simulink model "part1"  (R2020a)
settings: Solver=VariableStepAuto  StartTime=0.0  StopTime=3000  RelTol=1e-3
undefined symbols (not defined in the file): ConstSPSuge, ConstSPSway, ConstSPYaw, Current_input_type, Current_Speed, CurrHead, Hoerner, Kd_surge, Kd_sway, Kd_yaw, Ki_surge, Ki_sway, Ki_yaw, Kp_surge, Kp_sway, Kp_yaw, typeOfSimulation, vessel
libraries: marine_gnc x5, simulink x1, marine_hydro x1
settings Model: Creator=jonbjor  LastModifiedBy=joach
settings DataIOCC: ReturnWorkspaceOutputs=off
settings DebuggingCC: ArithmeticOperatorsInVariantConditions=warning
settings SFSimCC: SimUseLocalCustomCode=off  CustomCodeUndefinedFunction=UseInterfaceOnly
settings RTWCC: RTWUseLocalCustomCode=off

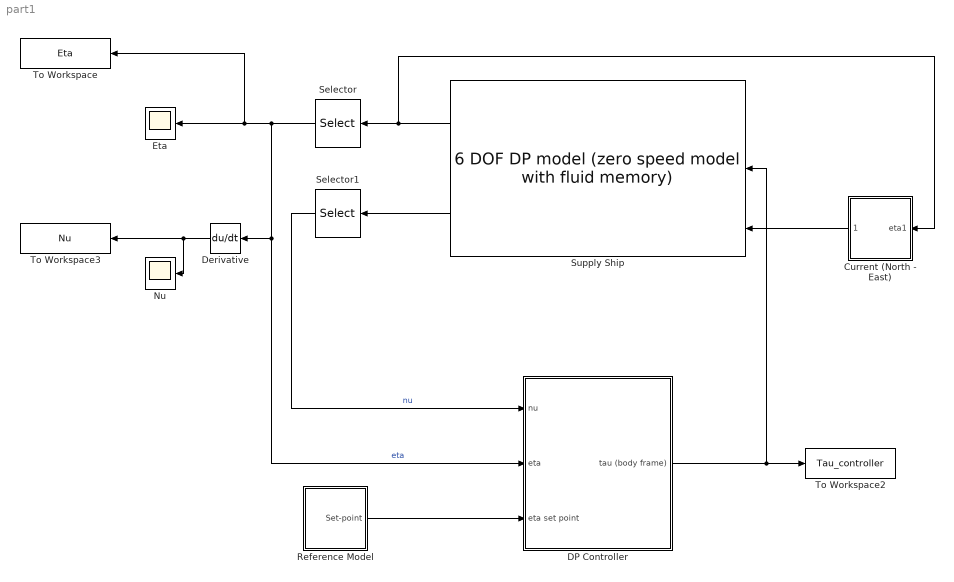
== system part1 ==
  Current (North - East) : Subsystem
  DP Controller : Subsystem
  Derivative : Derivative
  Eta : Scope
  Nu : Scope
  Reference Model : Subsystem
  Selector : Selector  InputPortWidth=6  IndexOptions=Index vector (dialog)  Indices=[1 2 6]  OutputSizes=1
  Selector1 : Selector  InputPortWidth=6  IndexOptions=Index vector (dialog)  Indices=[1 2 6]  OutputSizes=1
  Supply Ship : marine_hydro/Hydro Library/6 DOF DP model  (zero speed model with fluid memory)  ABC=vesselABC  rho=1025  Axc=0.9*vessel.main.T*vessel.main.B  Ayc=0.9*vessel.main.T*vessel.main.Lpp  CX=1  CY_2D=Hoerner(vessel.main.B,vessel.main.T)  Bv=vessel.Bv  mask(6 DOF zero speed model){}
      link override "Integrator1 ": InitialCondition=nu0
      link override Integrator2: InitialCondition=eta0
      settings: SourceProductName=MSS Hydro
      mask Display:
      | image('supply.jpg');
      | color('white'); port_label('output', 1, 'eta')
      | color('white'); port_label('output', 2, 'nu')
      | color('white'); port_label('input', 1, 'tau_wave')
      | color('white'); port_label('input', 2, 'tau')
      | color('white'); port_label('input', 3, 'nu_c')
  To Workspace : ToWorkspace  VariableName=Eta  SaveFormat=Timeseries  SampleTime=-1
  To Workspace2 : ToWorkspace  VariableName=Tau_controller  SaveFormat=Timeseries  SampleTime=-1
  To Workspace3 : ToWorkspace  VariableName=Nu  SaveFormat=Timeseries  SampleTime=-1
  wires:
  DP Controller/1(tau (body frame)) -> To Workspace2/1, Supply Ship/2
  Supply Ship/1 -> Current (North - East)/1(eta1), Selector/1
  Reference Model/1(Set-point) -> DP Controller/3(eta set point)
  Selector/1 -> Eta/1, To Workspace/1, DP Controller/2(eta), Derivative/1  "eta"
  Selector1/1 -> DP Controller/1(nu)  "nu"
  Current (North - East)/1(Current) -> Supply Ship/3
  Supply Ship/2 -> Selector1/1
  Derivative/1 -> Nu/1, To Workspace3/1

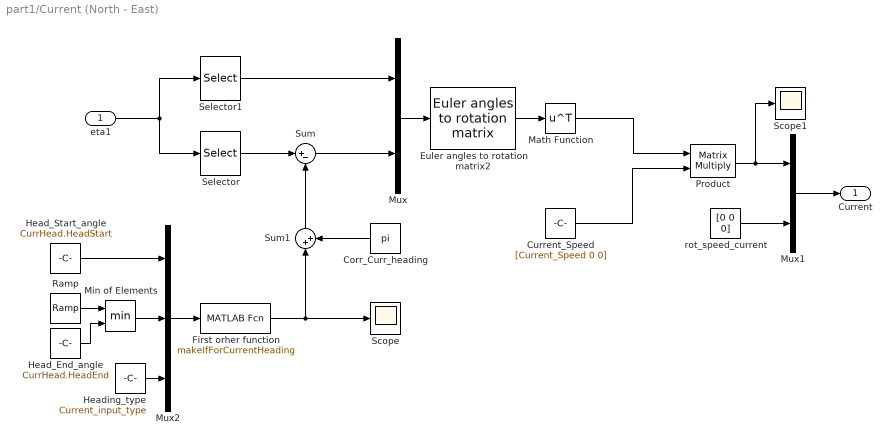
== system part1/Current (North - East) ==
  eta1 : Inport
  Corr_Curr_heading : Constant  Value=pi
  Current_Speed : Constant  Value=[Current_Speed 0 0]
  Euler angles to rotation matrix2 : marine_gnc/Models/ Kinematics/Euler angles to rotation matrix
      settings: SourceProductName=MSS GNC
  First orher function : MATLABFcn  MATLABFcn=makeIfForCurrentHeading
  Head_End_angle : Constant  Value=CurrHead.HeadEnd
  Head_Start_angle : Constant  Value=CurrHead.HeadStart
  Heading_type : Constant  Value=Current_input_type
  Math Function : Math  Operator=transpose  SaturateOnIntegerOverflow=on
  Min of Elements : MinMax  Inputs=2
  Mux : Mux  Inputs=2
  Mux1 : Mux  Inputs=2
  Mux2 : Mux  Inputs=3
  Product : Product  Inputs=**  Multiplication=Matrix(*)  SaturateOnIntegerOverflow=on  OutDataTypeStr=Inherit: Same as first input
  Ramp : simulink/Sources/Ramp  slope=CurrHead.Slope  start=CurrHead.TimeStart  InitialOutput=CurrHead.HeadStart
  Scope : Scope
  Scope1 : Scope
  Selector : Selector  InputPortWidth=6  IndexOptions=Index vector (dialog)  Indices=[6]  OutputSizes=1
  Selector1 : Selector  InputPortWidth=6  IndexOptions=Index vector (dialog)  Indices=[4 5]  OutputSizes=1
  Sum : Sum  Inputs=|+-
  Sum1 : Sum  Inputs=|++
  rot_speed_current : Constant  Value=[0 0 0]
  Current : Outport  VectorParamsAs1DForOutWhenUnconnected=off
  wires:
  Product/1 -> Scope1/1, Mux1/1
  eta1/1 -> Selector/1, Selector1/1
  Selector1/1 -> Mux/1
  Selector/1 -> Sum/1
  Sum/1 -> Mux/2
  Current_Speed/1 -> Product/2
  rot_speed_current/1 -> Mux1/2
  Mux1/1 -> Current/1
  Mux/1 -> Euler angles to rotation matrix2/1
  Euler angles to rotation matrix2/1 -> Math Function/1
  Math Function/1 -> Product/1
  Ramp/1 -> Min of Elements/1
  Head_End_angle/1 -> Min of Elements/2
  Head_Start_angle/1 -> Mux2/1
  Mux2/1 -> First orher function/1
  First orher function/1 -> Sum1/1, Scope/1
  Min of Elements/1 -> Mux2/2
  Heading_type/1 -> Mux2/3
  Corr_Curr_heading/1 -> Sum1/2
  Sum1/1 -> Sum/2

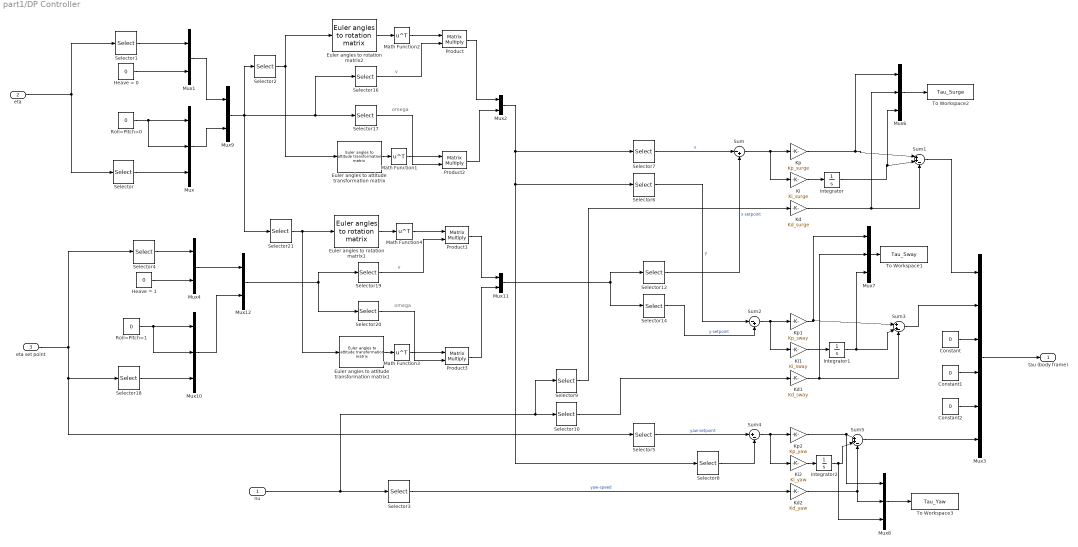
== system part1/DP Controller ==
  note: omega
  note: v
  note: omega
  note: v
  nu : Inport
  eta : Inport  Port=2
  eta set point : Inport  Port=3
  Constant : Constant  Value=0
  Constant1 : Constant  Value=0
  Constant2 : Constant  Value=0
  Euler angles to rotation matrix1 : marine_gnc/Models/ Kinematics/Euler angles to rotation matrix
      settings: SourceProductName=MSS GNC
  Euler angles to rotation matrix2 : marine_gnc/Models/ Kinematics/Euler angles to rotation matrix
      settings: SourceProductName=MSS GNC
  Euler angles to attitude transformation matrix : marine_gnc/Models/ Kinematics/Euler angles to attitude transformation matrix
      settings: SourceProductName=MSS GNC
  Euler angles to attitude transformation matrix1 : marine_gnc/Models/ Kinematics/Euler angles to attitude transformation matrix
      settings: SourceProductName=MSS GNC
  Heave = 0 : Constant  Value=0
  Heave = 1 : Constant  Value=0
  Integrator : Integrator
  Integrator1 : Integrator
  Integrator2 : Integrator
  Kd : Gain  Gain=Kd_surge
  Kd1 : Gain  Gain=Kd_sway
  Kd2 : Gain  Gain=Kd_yaw
  Ki : Gain  Gain=Ki_surge
  Ki1 : Gain  Gain=Ki_sway
  Ki2 : Gain  Gain=Ki_yaw
  Kp : Gain  Gain=Kp_surge
  Kp1 : Gain  Gain=Kp_sway
  Kp2 : Gain  Gain=Kp_yaw
  Math Function{1..4} (4 alike) : Math  Operator=transpose  SaturateOnIntegerOverflow=on
  Mux{,6..8,10} (5 alike) : Mux  Inputs=3
  Mux{1..2,4,9,11..12} (6 alike) : Mux  Inputs=2
  Mux3 : Mux  Inputs=6
  Product{,1..3} (4 alike) : Product  Inputs=**  Multiplication=Matrix(*)  SaturateOnIntegerOverflow=on  OutDataTypeStr=Inherit: Same as first input
  Roll=Pitch=0 : Constant  Value=0
  Roll=Pitch=1 : Constant  Value=0
  Selector : Selector  InputPortWidth=3  IndexOptions=Index vector (dialog)  Indices=[3]  OutputSizes=1
  Selector1 : Selector  InputPortWidth=3  IndexOptions=Index vector (dialog)  Indices=[1 2]  OutputSizes=1
  Selector10 : Selector  InputPortWidth=3  IndexOptions=Index vector (dialog)  Indices=2  OutputSizes=1
  Selector12 : Selector  InputPortWidth=6  IndexOptions=Index vector (dialog)  Indices=1  OutputSizes=1
  Selector14 : Selector  InputPortWidth=6  IndexOptions=Index vector (dialog)  Indices=2  OutputSizes=1
  Selector16 : Selector  InputPortWidth=6  IndexOptions=Index vector (dialog)  Indices=[1 2 3]  OutputSizes=1
  Selector{2,17,20..21} (4 alike) : Selector  InputPortWidth=6  IndexOptions=Index vector (dialog)  Indices=[4 5 6]  OutputSizes=1
  Selector18 : Selector  InputPortWidth=3  IndexOptions=Index vector (dialog)  Indices=[3]  OutputSizes=1
  Selector19 : Selector  InputPortWidth=6  IndexOptions=Index vector (dialog)  Indices=[1 2 3]  OutputSizes=1
  Selector3 : Selector  InputPortWidth=3  IndexOptions=Index vector (dialog)  Indices=3  OutputSizes=1
  Selector4 : Selector  InputPortWidth=3  IndexOptions=Index vector (dialog)  Indices=[1 2]  OutputSizes=1
  Selector5 : Selector  InputPortWidth=3  IndexOptions=Index vector (dialog)  Indices=[3]  OutputSizes=1
  Selector6 : Selector  InputPortWidth=6  IndexOptions=Index vector (dialog)  Indices=2  OutputSizes=1
  Selector7 : Selector  InputPortWidth=6  IndexOptions=Index vector (dialog)  Indices=1  OutputSizes=1
  Selector8 : Selector  InputPortWidth=6  IndexOptions=Index vector (dialog)  Indices=[6]  OutputSizes=1
  Selector9 : Selector  InputPortWidth=3  IndexOptions=Index vector (dialog)  Indices=1  OutputSizes=1
  Sum : Sum  Inputs=|-+
  Sum1 : Sum  Inputs=|++-
  Sum2 : Sum  Inputs=|-+
  Sum3 : Sum  Inputs=|++-
  Sum4 : Sum  Inputs=|+-
  Sum5 : Sum  Inputs=|++-
  To Workspace1 : ToWorkspace  VariableName=Tau_Sway  SaveFormat=Timeseries  SampleTime=-1
  To Workspace2 : ToWorkspace  VariableName=Tau_Surge  SaveFormat=Timeseries  SampleTime=-1
  To Workspace3 : ToWorkspace  VariableName=Tau_Yaw  SaveFormat=Timeseries  SampleTime=-1
  tau (body frame) : Outport  VectorParamsAs1DForOutWhenUnconnected=off
  wires:
  Roll=Pitch=0/1 -> Mux/1, Mux/2
  Selector7/1 -> Sum/1  "x"
  Selector12/1 -> Sum/2  "x-setpoint"
  Sum/1 -> Ki/1, Kp/1
  Kp/1 -> Mux6/1, Sum1/1
  Integrator/1 -> Mux6/3, Sum1/2
  Kd/1 -> Mux6/2, Sum1/3
  Kp1/1 -> Mux7/1, Sum3/1
  Sum2/1 -> Ki1/1, Kp1/1
  Integrator1/1 -> Sum3/2, Mux7/3
  Selector6/1 -> Sum2/1  "y"
  Kd1/1 -> Mux7/2, Sum3/3
  Selector14/1 -> Sum2/2  "y-setpoint"
  Integrator2/1 -> Mux8/3, Sum5/2
  Sum4/1 -> Ki2/1, Kp2/1
  Sum5/1 -> Mux3/6
  Kp2/1 -> Mux8/1, Sum5/1
  Kd2/1 -> Mux8/2, Sum5/3
  Selector/1 -> Mux/3
  Selector5/1 -> Sum4/1  "yaw-setpoint"
  Constant/1 -> Mux3/3
  Constant1/1 -> Mux3/4
  Constant2/1 -> Mux3/5
  Selector1/1 -> Mux1/1
  Heave = 0/1 -> Mux1/2
  Mux11/1 -> Selector14/1, Selector12/1
  Selector4/1 -> Mux4/1
  Heave = 1/1 -> Mux4/2
  Sum1/1 -> Mux3/1
  Ki/1 -> Integrator/1
  Ki1/1 -> Integrator1/1
  Ki2/1 -> Integrator2/1
  Sum3/1 -> Mux3/2
  Selector3/1 -> Kd2/1  "yaw-speed"
  nu/1 -> Selector9/1, Selector10/1, Selector3/1
  Selector9/1 -> Kd/1
  Selector10/1 -> Kd1/1
  Selector8/1 -> Sum4/2
  Mux3/1 -> tau (body frame)/1
  Mux6/1 -> To Workspace2/1
  Mux7/1 -> To Workspace1/1
  Mux8/1 -> To Workspace3/1
  eta/1 -> Selector/1, Selector1/1
  Selector16/1 -> Product/2
  Selector2/1 -> Euler angles to attitude transformation matrix/1, Euler angles to rotation matrix2/1
  Euler angles to rotation matrix2/1 -> Math Function2/1
  Euler angles to attitude transformation matrix/1 -> Math Function1/1
  Product2/1 -> Mux2/2
  Selector17/1 -> Product2/2
  Product/1 -> Mux2/1
  Mux1/1 -> Mux9/1
  Math Function1/1 -> Product2/1
  Math Function2/1 -> Product/1
  Mux/1 -> Mux9/2
  Mux9/1 -> Selector21/1, Selector2/1, Selector17/1, Selector16/1
  Mux2/1 -> Selector6/1, Selector8/1, Selector7/1
  eta set point/1 -> Selector4/1, Selector18/1, Selector5/1
  Roll=Pitch=1/1 -> Mux10/1, Mux10/2
  Selector18/1 -> Mux10/3
  Euler angles to rotation matrix1/1 -> Math Function4/1
  Product3/1 -> Mux11/2
  Euler angles to attitude transformation matrix1/1 -> Math Function3/1
  Mux12/1 -> Selector20/1, Selector19/1
  Math Function4/1 -> Product1/1
  Selector19/1 -> Product1/2
  Selector21/1 -> Euler angles to rotation matrix1/1, Euler angles to attitude transformation matrix1/1
  Math Function3/1 -> Product3/1
  Selector20/1 -> Product3/2
  Mux4/1 -> Mux12/1
  Product1/1 -> Mux11/1
  Mux10/1 -> Mux12/2

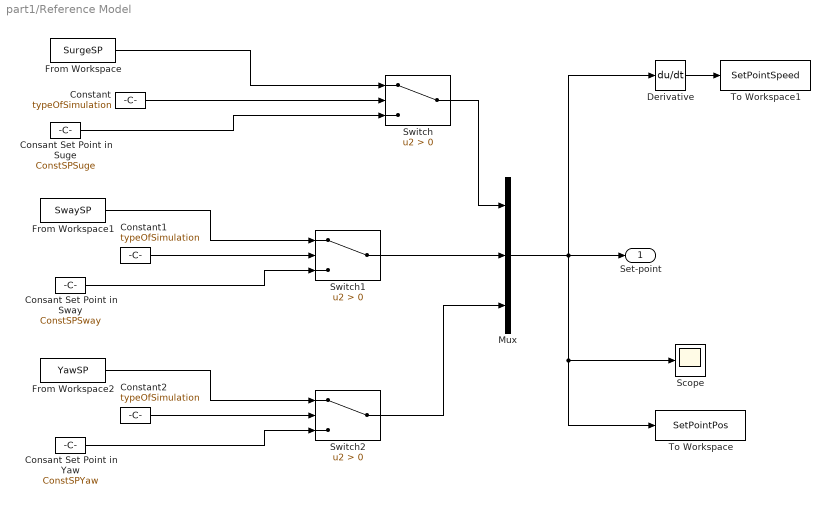
== system part1/Reference Model ==
  Consant Set Point in Suge : Constant  Value=ConstSPSuge
  Consant Set Point in Sway : Constant  Value=ConstSPSway
  Consant Set Point in Yaw : Constant  Value=ConstSPYaw
  Constant : Constant  Value=typeOfSimulation
  Constant1 : Constant  Value=typeOfSimulation
  Constant2 : Constant  Value=typeOfSimulation
  Derivative : Derivative
  From Workspace : FromWorkspace  VariableName=SurgeSP
  From Workspace1 : FromWorkspace  VariableName=SwaySP
  From Workspace2 : FromWorkspace  VariableName=YawSP
  Mux : Mux  Inputs=3
  Scope : Scope
  Switch : Switch  Criteria=u2 > Threshold
  Switch1 : Switch  Criteria=u2 > Threshold
  Switch2 : Switch  Criteria=u2 > Threshold
  To Workspace : ToWorkspace  VariableName=SetPointPos  SaveFormat=Timeseries  SampleTime=-1
  To Workspace1 : ToWorkspace  VariableName=SetPointSpeed  SaveFormat=Timeseries  SampleTime=-1
  Set-point : Outport  VectorParamsAs1DForOutWhenUnconnected=off
  wires:
  Switch/1 -> Mux/1
  Constant/1 -> Switch/2
  Consant Set Point in Suge/1 -> Switch/3
  From Workspace1/1 -> Switch1/1
  Consant Set Point in Sway/1 -> Switch1/3
  Constant1/1 -> Switch1/2
  Switch1/1 -> Mux/2
  Switch2/1 -> Mux/3
  Consant Set Point in Yaw/1 -> Switch2/3
  From Workspace2/1 -> Switch2/1
  Constant2/1 -> Switch2/2
  From Workspace/1 -> Switch/1
  Mux/1 -> Derivative/1, To Workspace/1, Scope/1, Set-point/1
  Derivative/1 -> To Workspace1/1
